simulink model "PIDcontrol"  (R2019b)
settings: Solver=VariableStepAuto  StartTime=0.0  StopTime=SimulationTime  RelTol=1e-3
values from neighbouring files (symbols this model uses):
  D = 0.075    [Obliczenia.m]
  D2 = 0.075    [Obliczenia.m]
  disturbanceStrength = 0.001    [Obliczenia.m]
  I = 0.2    [Obliczenia.m]
  I2 = 0.2    [Obliczenia.m]
  kd = delay    (= 1)    [Obliczenia.m]
  lambda = 0.05    [Obliczenia.m]
  N = 1    [Obliczenia.m]
  objDen = [-1.1 0.3 0]    [Obliczenia.m]
  objDen2 = [-1.1 0.3 -0.15]    [Obliczenia.m]
  objNum = [0.75 0.5 0 0]    [Obliczenia.m]
  objNum2 = [0.75 0.5 0 0]    [Obliczenia.m]
  P = 0.84    [Obliczenia.m]
  P2 = 0.84    [Obliczenia.m]
  RegulatedValue = 5    [Obliczenia.m]
  SampleTime = 1    [Obliczenia.m]
libraries: simulink x6
settings Model: Creator=pleka  LastModifiedBy=pleka

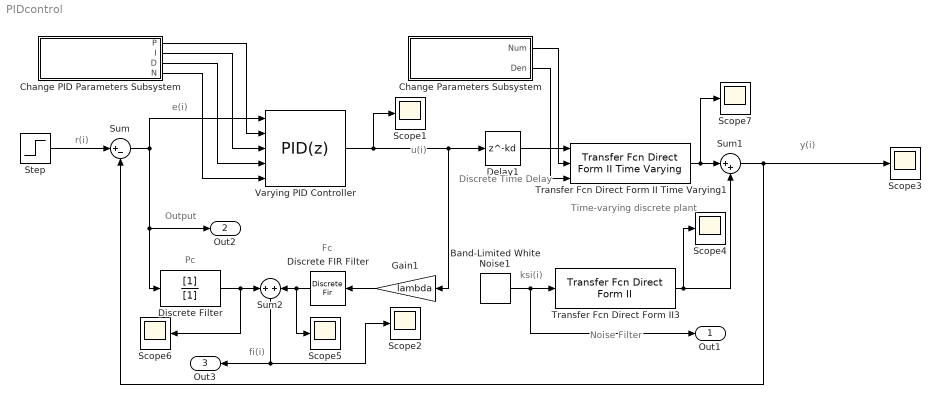
== system PIDcontrol ==
  note: Pc
  note: Fc
  note: fi(i)
  note: e(i)
  note: Discrete Time Delay
  note: ksi(i)
  note: Output
  note: u(i)
  note: y(i)
  note: Noise Filter
  note: r(i)
  note: Time-varying discrete plant
  Band-Limited White Noise1 : simulink/Sources/Band-Limited White Noise  Cov=[disturbanceStrength]  Ts=SampleTime  seed=[23341]
  Change PID Parameters Subsystem : Subsystem
  Change Parameters Subsystem : Subsystem
  Delay1 : Delay  DelayLength=kd
  Discrete FIR Filter : DiscreteFir  Coefficients=[1]
  Discrete Filter : DiscreteFilter  Denominator=[1]
  Gain1 : Gain  Gain=lambda
  Scope{1..7} (7 alike) : Scope
  Step : Step  Time=0  After=RegulatedValue  SampleTime=SampleTime
  Sum : Sum  Inputs=|+-
  Sum1 : Sum  Inputs=|++
  Sum2 : Sum  Inputs=+|+
  Transfer Fcn Direct Form II Time Varying1 : simulink/Additional Math & Discrete/Additional Discrete/Transfer Fcn Direct Form II Time Varying  vinit=0.0  DoSatur=off
      settings: SourceProductName=Simulink  SourceProductBaseCode=SL
  Transfer Fcn Direct Form II3 : simulink/Additional Math & Discrete/Additional Discrete/Transfer Fcn Direct Form II  NumCoefVec=errorNum  DenCoefVec=errorDen  vinit=0.0  DoSatur=off
      settings: SourceProductName=Simulink  SourceProductBaseCode=SL
  Varying PID Controller : simulink/Continuous/PID Controller  Controller=PID  Form=Parallel  TimeDomain=Discrete-time  SampleTime=SampleTime  IntegratorMethod=Forward Euler  FilterMethod=Forward Euler  ControllerParametersSource=external  P=1  I=1  D=0  UseFilter=on  N=100  TunerSelectOption=Transfer Function Based (PID Tuner App)  InitialConditionSource=internal  InitialConditionForIntegrator=0  InitialConditionForFilter=0  DifferentiatorICPrevScaledInput=0  ExternalReset=none  TrackingMode=off  Kt=1  LimitOutput=off  UpperSaturationLimit=inf  LowerSaturationLimit=-inf  LinearizeAsGain=on  AntiWindupMode=none  Kb=1  POutMin=[]  POutMax=[]  IOutMin=[]  IOutMax=[]  DOutMin=[]  DOutMax=[]  NOutMin=[]  NOutMax=[]  SumOutMin=[]  SumOutMax=[]  SaturationOutMin=[]  SaturationOutMax=[]  PParamMin=[]  PParamMax=[]  IParamMin=[]  IParamMax=[]  DParamMin=[]  DParamMax=[]  NParamMin=[]  NParamMax=[]  KbParamMin=[]  KbParamMax=[]  KtParamMin=[]  KtParamMax=[]  KbOutMin=[]  KbOutMax=[]  KtOutMin=[]  KtOutMax=[]  IntegratorOutMin=[]  IntegratorOutMax=[]  FilterOutMin=[]  FilterOutMax=[]  SumI1OutMin=[]  SumI1OutMax=[]  SumI2OutMin=[]  SumI2OutMax=[]  SumI3OutMin=[]  SumI3OutMax=[]  SumI4OutMin=[]  SumI4OutMax=[]  SumDOutMin=[]  SumDOutMax=[]  DifferentiatorOutMin=[]  DifferentiatorOutMax=[]  FilterDiffOutCoefMin=[]  FilterDiffOutCoefMax=[]  ReciprocalOutMin=[]  ReciprocalOutMax=[]  SumDenOutMin=[]  SumDenOutMax=[]  SumNumOutMin=[]  SumNumOutMax=[]  DivideOutMin=[]  DivideOutMax=[]  IntegratorContinuousStateAttributes=''  IntegratorStateMustResolveToSignalObject=off  IntegratorRTWStateStorageClass=Auto  FilterContinuousStateAttributes=''  FilterStateMustResolveToSignalObject=off  FilterRTWStateStorageClass=Auto  ParallelPVariant=ExternalParameters  IdealPVariant=Disabled  IVariant=ExternalParameters  DVariant=ExternalParameters  IntegratorVariant=Discrete  SatVariant=Disabled  AWVariant=Passthrough  PCopyVariant=Disabled  TRVariant=Disabled  FdbkBlocksVariant=Forward  IdealPFdbkVariant=Disabled  SatFdbkVariant=Disabled  DerivativeFilterVariant=ForwardEulerFilter  NVariant=ExternalParameters  NCopyVariant=Disabled  FilterICVariant=InternalICsFilter  IntegratorICVariant=InternalICs  ExternalResetVariant=Disabled  TRSumVariant=Passthrough  SumFdbkVariant=Disabled  SumVariant=Sum_PID
  Out1 : Outport
  Out2 : Outport  Port=2
  Out3 : Outport  Port=3
  wires:
  Sum1/1 -> Sum/2, Scope3/1
  Band-Limited White Noise1/1 -> Out1/1, Transfer Fcn Direct Form II3/1
  Transfer Fcn Direct Form II3/1 -> Sum1/2, Scope4/1
  Change Parameters Subsystem/1(Num) -> Transfer Fcn Direct Form II Time Varying1/2
  Change Parameters Subsystem/2(Den) -> Transfer Fcn Direct Form II Time Varying1/3
  Transfer Fcn Direct Form II Time Varying1/1 -> Scope7/1, Sum1/1
  Step/1 -> Sum/1
  Varying PID Controller/1 -> Scope1/1, Delay1/1, Gain1/1
  Change PID Parameters Subsystem/1(P) -> Varying PID Controller/2
  Change PID Parameters Subsystem/2(I) -> Varying PID Controller/3
  Change PID Parameters Subsystem/3(D) -> Varying PID Controller/4
  Change PID Parameters Subsystem/4(N) -> Varying PID Controller/5
  Sum/1 -> Discrete Filter/1, Out2/1, Varying PID Controller/1
  Gain1/1 -> Discrete FIR Filter/1
  Discrete Filter/1 -> Scope6/1, Sum2/1
  Discrete FIR Filter/1 -> Scope5/1, Sum2/2
  Sum2/1 -> Scope2/1, Out3/1
  Delay1/1 -> Transfer Fcn Direct Form II Time Varying1/1

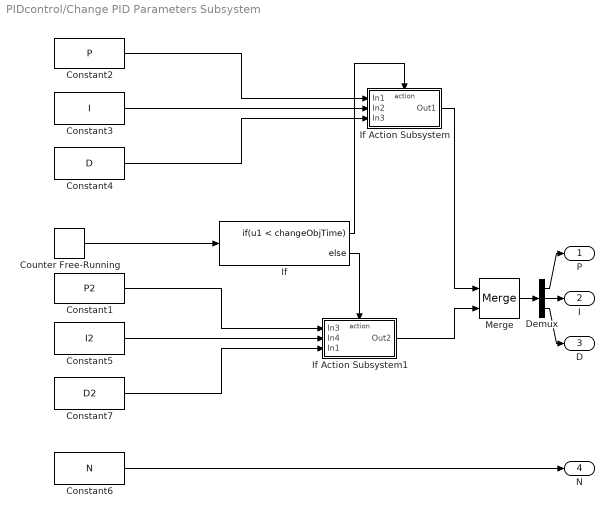
== system PIDcontrol/Change PID Parameters Subsystem ==
  Constant1 : Constant  Value=P2
  Constant2 : Constant  Value=P
  Constant3 : Constant  Value=I
  Constant4 : Constant  Value=D
  Constant5 : Constant  Value=I2
  Constant6 : Constant  Value=N
  Constant7 : Constant  Value=D2
  Counter Free-Running : simulink/Sources/Counter Free-Running  NumBits=16  tsamp=-1
  Demux : Demux  Outputs=3
  If : If  IfExpression=u1 < changeObjTime
  If Action Subsystem : Subsystem  TreatAsAtomicUnit=on
  If Action Subsystem1 : Subsystem  TreatAsAtomicUnit=on
  Merge : Merge
  P : Outport
  I : Outport  Port=2
  D : Outport  Port=3
  N : Outport  Port=4
  wires:
  Counter Free-Running/1 -> If/1
  If/2 -> If Action Subsystem1/Action
  If/1 -> If Action Subsystem/Action
  Constant3/1 -> If Action Subsystem/2(In2)
  Constant2/1 -> If Action Subsystem/1(In1)
  Constant6/1 -> N/1
  Merge/1 -> Demux/1
  Demux/1 -> P/1
  Demux/2 -> I/1
  Demux/3 -> D/1
  Constant4/1 -> If Action Subsystem/3(In3)
  If Action Subsystem/1(Out1) -> Merge/1
  Constant5/1 -> If Action Subsystem1/2(In4)
  Constant1/1 -> If Action Subsystem1/1(In3)
  Constant7/1 -> If Action Subsystem1/3(In1)
  If Action Subsystem1/1(Out2) -> Merge/2

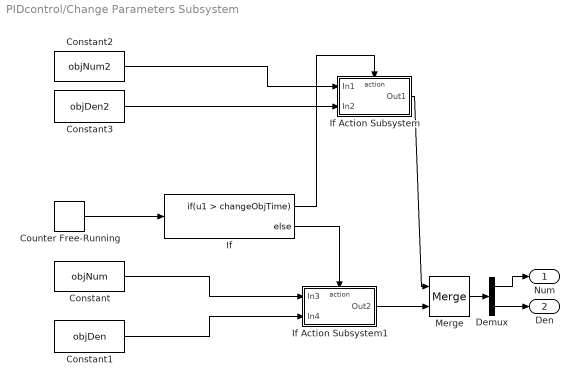
== system PIDcontrol/Change Parameters Subsystem ==
  Constant : Constant  Value=objNum
  Constant1 : Constant  Value=objDen
  Constant2 : Constant  Value=objNum2
  Constant3 : Constant  Value=objDen2
  Counter Free-Running : simulink/Sources/Counter Free-Running  NumBits=16  tsamp=-1
  Demux : Demux  Outputs=2
  If : If  IfExpression=u1 > changeObjTime
  If Action Subsystem : Subsystem  TreatAsAtomicUnit=on
  If Action Subsystem1 : Subsystem  TreatAsAtomicUnit=on
  Merge : Merge
  Num : Outport
  Den : Outport  Port=2
  wires:
  Counter Free-Running/1 -> If/1
  If/2 -> If Action Subsystem1/Action
  If/1 -> If Action Subsystem/Action
  Constant3/1 -> If Action Subsystem/2(In2)
  Constant2/1 -> If Action Subsystem/1(In1)
  Merge/1 -> Demux/1
  Constant/1 -> If Action Subsystem1/1(In3)
  Constant1/1 -> If Action Subsystem1/2(In4)
  If Action Subsystem/1(Out1) -> Merge/1
  If Action Subsystem1/1(Out2) -> Merge/2
  Demux/1 -> Num/1
  Demux/2 -> Den/1

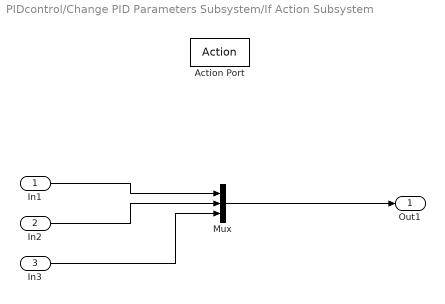
== system PIDcontrol/Change PID Parameters Subsystem/If Action Subsystem ==
  In1 : Inport
  In2 : Inport  Port=2
  In3 : Inport  Port=3
  Action Port : ActionPort  ActionPortLabel=if(u1 < changeObjTime)
  Mux : Mux  Inputs=3
  Out1 : Outport
  wires:
  Mux/1 -> Out1/1
  In1/1 -> Mux/1
  In2/1 -> Mux/2
  In3/1 -> Mux/3

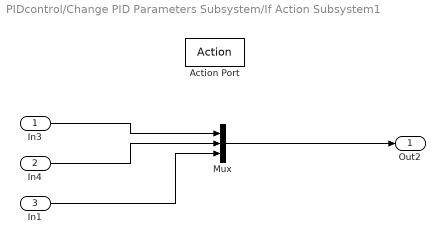
== system PIDcontrol/Change PID Parameters Subsystem/If Action Subsystem1 ==
  In3 : Inport
  In4 : Inport  Port=2
  In1 : Inport  Port=3
  Action Port : ActionPort  ActionPortLabel=else
  Mux : Mux  Inputs=3
  Out2 : Outport
  wires:
  In4/1 -> Mux/2
  In3/1 -> Mux/1
  Mux/1 -> Out2/1
  In1/1 -> Mux/3

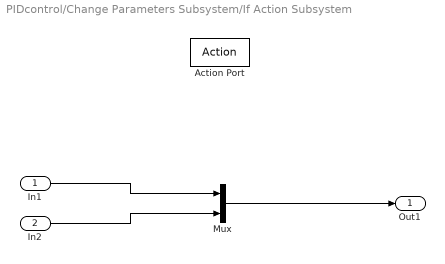
== system PIDcontrol/Change Parameters Subsystem/If Action Subsystem ==
  In1 : Inport
  In2 : Inport  Port=2
  Action Port : ActionPort  ActionPortLabel=if(u1 > changeObjTime)
  Mux : Mux  Inputs=2
  Out1 : Outport
  wires:
  Mux/1 -> Out1/1
  In1/1 -> Mux/1
  In2/1 -> Mux/2

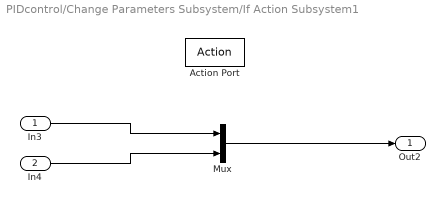
== system PIDcontrol/Change Parameters Subsystem/If Action Subsystem1 ==
  In3 : Inport
  In4 : Inport  Port=2
  Action Port : ActionPort  ActionPortLabel=else
  Mux : Mux  Inputs=2
  Out2 : Outport
  wires:
  In4/1 -> Mux/2
  In3/1 -> Mux/1
  Mux/1 -> Out2/1
